simulink model "vf_ann_model"  (R2024a)
settings: Solver=ode3  StartTime=0.0  StopTime=30  FixedStep=1e-5  RelTol=1e-3
libraries: spsIGBTDiodeLib x6, spsCurrentMeasurementLib x3, spsAsynchronousMachineSIUnitsLib x1, spsDCVoltageSourceLib x1, simulink x1, sps_lib x1
settings Model: Creator=vani1  LastModifiedBy=vani1

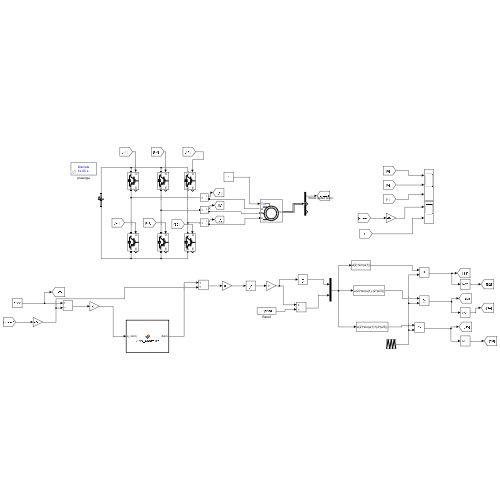
[thumbnail: Simulink's stored preview of the top-level diagram]
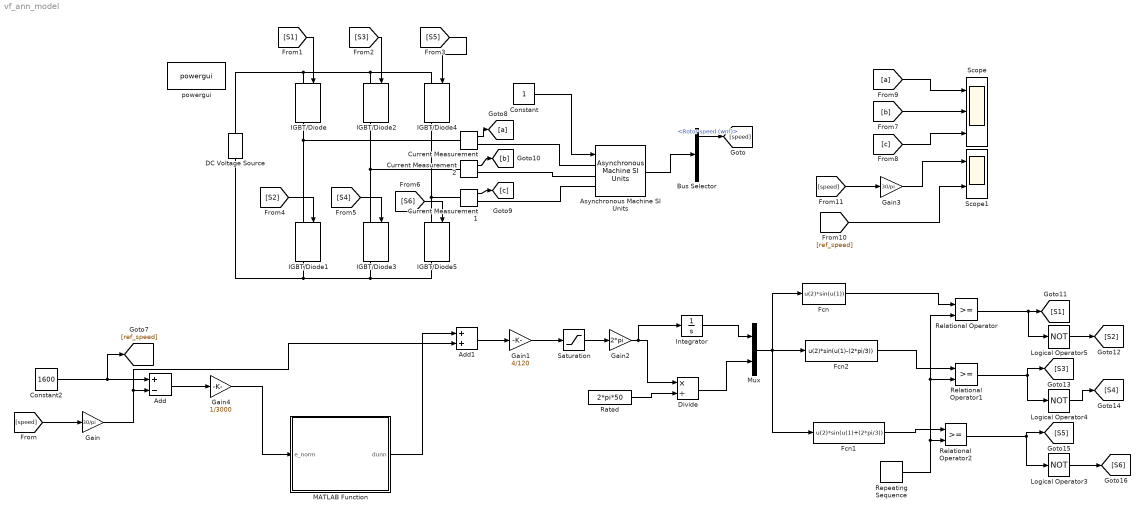
== system vf_ann_model ==
  Add : Sum  Inputs=+-
  Add1 : Sum
  Asynchronous Machine SI Units : spsAsynchronousMachineSIUnitsLib/Asynchronous Machine SI Units  RotorType=Squirrel-cage  PresetModel=No  MechanicalLoad=Torque Tm  ShowDetailedParameters=on  ReferenceFrame=Rotor  Units=SI  MeasurementBus=off  NominalParameters=[1.845e+04 400 50]  VoltageRatio=1  Stator=[0.5968 0.0003495]  Rotor=[0.6258 0.005473]  Cage1=[0.4155 0.002066]  Cage2=[0.4168 0.0003495]  Lm=0.0354  Mechanical=[0.05 0.005879 2]  PolePairs=2  InitialConditions=[0 0 0 0 0 0 0 0]  SimulateSaturation=off  Saturation=[14.03593122, 27.81365428, 53.79336849, 72.68890987, 97.98006896, 148.6815601, 215.7428561, 302.9841135, 428.7778367 ; 230, 322, 414, 460, 506, 552, 598, 644, 690]  LoadFlowParameters=1492000  TsPowergui=0  TsBlock=-1  IterativeModel=Trapezoidal non iterative  IterativeDiscreteModel=Trapezoidal non iterative  Pmec=1.492e+006
  Bus Selector : BusSelector  OutputSignals=Mechanical.Rotor speed (wm),Mechanical.Rotor angle thetam (rad),Mechanical.Electromagnetic torque Te (N*m)
  Constant : Constant
  Constant2 : Constant  Value=1600
  Current Measurement : spsCurrentMeasurementLib/Current Measurement  PhasorSimulation=off  OutputType=Complex  PSBequivalent=0
  Current Measurement1 : spsCurrentMeasurementLib/Current Measurement  PhasorSimulation=off  OutputType=Complex  PSBequivalent=0
  Current Measurement2 : spsCurrentMeasurementLib/Current Measurement  PhasorSimulation=off  OutputType=Complex  PSBequivalent=0
  DC Voltage Source : spsDCVoltageSourceLib/DC Voltage Source  Amplitude=650  Measurements=None
  Divide : Product  Inputs=*/
  Fcn : Fcn  Expr=u(2)*sin(u(1))
  Fcn1 : Fcn  Expr=u(2)*sin(u(1)+(2*pi/3))
  Fcn2 : Fcn  Expr=u(2)*sin(u(1)-(2*pi/3))
  Gain : Gain  Gain=30/pi
  Gain1 : Gain  Gain=4/120
  Gain2 : Gain  Gain=2*pi
  Gain3 : Gain  Gain=30/pi
  Gain4 : Gain  Gain=1/3000
  IGBT/Diode{,1..5} (6 alike) : spsIGBTDiodeLib/IGBT//Diode  Ron=1e-3  Rs=1e5  Cs=inf  Measurements=on
  Integrator : Integrator
  Logical Operator3 : Logic  Operator=NOT  AllPortsSameDT=off  OutDataTypeStr=boolean
  Logical Operator4 : Logic  Operator=NOT  AllPortsSameDT=off  OutDataTypeStr=boolean
  Logical Operator5 : Logic  Operator=NOT  AllPortsSameDT=off  OutDataTypeStr=boolean
  MATLAB Function : MATLAB Function  TreatAsAtomicUnit=on
  Mux : Mux  Inputs=2
  Rated : Constant  Value=2*pi*50
  Relational Operator : RelationalOperator  OutDataTypeStr=boolean  RndMeth=Simplest  InputSameDT=off
  Relational Operator1 : RelationalOperator  OutDataTypeStr=boolean  RndMeth=Simplest  InputSameDT=off
  Relational Operator2 : RelationalOperator  OutDataTypeStr=boolean  RndMeth=Simplest  InputSameDT=off
  Repeating Sequence : simulink/Sources/Repeating Sequence  rep_seq_t=[0 1 2]*(1/5000)  rep_seq_y=[-1 1 -1]
  Saturation : Saturate  UpperLimit=100  LowerLimit=0
  Scope : Scope  NumInputPorts=3
  Scope1 : Scope  NumInputPorts=2
  powergui : sps_lib/powergui  Priority=1  SimulationMode=Discrete  SampleTime=1e-5  frequency=60  Iterations=50  frequencyindice=50  Pbase=100e6  ErrMax=1e-4  UnitsV=kV  UnitsW=MW  buscounter=0  FunctionMessages=off  echomessages=off  EnableUseOfTLC=off  CurrentSourceSwitches=off  DisableSnubberDevices=off  DisableRonSwitches=off  DisableVfSwitches=off  DisplayEquations=off  AutomaticDiscreteSolvers=off  SolverType=Tustin  Interpol=off  ExternalGateDelay=off  methode=off  Ts=100  x0status=blocks  SPID=on  SwTol=0  HookPort=off  NonlinearTolerance=1e-4  nMaxIteration=100  ContinueOnMaxIteration=off  RestoreLinks=warning  ResistiveCurrentMeasurement=off  Frange=[0:2:500]  Ylog=off  Xlog=on  ShowGrid=off  save=off  variable=ZData  structure=0  ZoomFFT=off  StartTime=0.0  cycles=1  DisplayStyle=1  fundamental=60  FreqAxis=off  MaxFrequency=1000  frequencyindicesteady=1  RmsSteady=1  display=off
  wires:
  Constant/1 -> Asynchronous Machine SI Units/1
  Asynchronous Machine SI Units/1 -> Bus Selector/1
  Bus Selector/1 -> [speed]  "<Rotor speed (wm)>"
  [speed] -> Gain/1
  Gain/1 -> Add1/2, Add/2
  Add/1 -> Gain4/1
  Gain1/1 -> Saturation/1
  Saturation/1 -> Gain2/1
  Gain2/1 -> Divide/1, Integrator/1
  Rated/1 -> Divide/2
  Divide/1 -> Mux/2
  Mux/1 -> Fcn/1, Fcn2/1, Fcn1/1
  [S1] -> IGBT/Diode/1
  [S2] -> IGBT/Diode1/1
  [S4] -> IGBT/Diode3/1
  [S6] -> IGBT/Diode5/1
  Current Measurement/1 -> [a]
  Current Measurement2/1 -> [b]
  Current Measurement1/1 -> [c]
  [c] -> Scope/3
  [a] -> Scope/1
  [b] -> Scope/2
  [speed] -> Gain3/1
  Gain3/1 -> Scope1/1
  [ref_speed] -> Scope1/2
  Integrator/1 -> Mux/1
  Fcn/1 -> Relational Operator/1
  Fcn2/1 -> Relational Operator1/1
  Fcn1/1 -> Relational Operator2/1
  Relational Operator/1 -> Logical Operator5/1, [S1]
  Logical Operator5/1 -> [S2]
  Relational Operator1/1 -> Logical Operator4/1, [S3]
  Logical Operator4/1 -> [S4]
  Relational Operator2/1 -> Logical Operator3/1, [S5]
  Logical Operator3/1 -> [S6]
  Repeating Sequence/1 -> Relational Operator2/2, Relational Operator1/2, Relational Operator/2
  Add1/1 -> Gain1/1
  [S3] -> IGBT/Diode2/1
  [S5] -> IGBT/Diode4/1
  Constant2/1 -> [ref_speed], Add/1
  MATLAB Function/1(dunn) -> Add1/1
  Gain4/1 -> MATLAB Function/1(e_norm)
  connections:
  IGBT/Diode1/LConn1 -- Current Measurement/LConn1 -- IGBT/Diode/RConn1
  IGBT/Diode3/LConn1 -- Current Measurement2/LConn1 -- IGBT/Diode2/RConn1
  IGBT/Diode5/LConn1 -- IGBT/Diode4/RConn1 -- Current Measurement1/LConn1
  IGBT/Diode/LConn1 -- DC Voltage Source/RConn1 -- IGBT/Diode4/LConn1 -- IGBT/Diode2/LConn1
  IGBT/Diode1/RConn1 -- DC Voltage Source/LConn1 -- IGBT/Diode5/RConn1 -- IGBT/Diode3/RConn1
  Current Measurement/RConn1 -- Asynchronous Machine SI Units/LConn1
  Current Measurement2/RConn1 -- Asynchronous Machine SI Units/LConn2
  Current Measurement1/RConn1 -- Asynchronous Machine SI Units/LConn3

== matlab function vf_ann_model/MATLAB Function ==
  data: e_norm input; dunn output
function dunn = ANN_Controller(e_norm)
    %#codegen
    persistent w1 w2 w3 loaded

    if isempty(loaded)
        s = load('ann_weights.mat');
        w1 = s.w1;
        w2 = s.w2;
        w3 = s.w3;
        loaded = true;
    end

    a1 = tanh(w1 * e_norm);
    a2 = tanh(w2 * a1);
    dunn = w3 * a2;
end
